simulink model "PlantaSoloActitud"  (Simulink 8.0)
settings: Solver=ode4  StartTime=0.0  StopTime=inf  FixedStep=0.001  RelTol=1e-3
undefined symbols (not defined in the file or in its folder): PlantaActitudOneStepMOD, VEFI_to_VE
libraries: simulink x3
settings Model: Creator=alumno4  LastModifiedBy=David  ExtModeTrigDuration=5000
settings SolverCC: PositivePriorityOrder=on
settings DataIOCC: SignalLoggingSaveFormat=ModelDataLogs
settings OptimizationCC: InlineParams=on
settings DebuggingCC: FcnCallInpInsideContextMsg=UseLocalSettings
settings RTWCC: SystemTargetFile=quarc_windows.tlc  TemplateMakefile=quarc_default_tmf  Description=QUARC Win32 Target  ProcessScript=quarc_windows_make_rtw_hook
settings STFCustomTargetCC: TargetPreCompLibLocation=C:\PROGRA~2\QUARC\lib\2011a\windows\release  CodeReplacementLibrary=ANSI_C  GeneratePreprocessorConditionals=Disable all  SystemTargetFile=quarc_windows.tlc
settings GRTTargetCC: TargetPreCompLibLocation=C:\PROGRA~2\QUARC\lib\2011a\windows\release  ParMdlRefBuildCompliant=off  CompOptLevelCompliant=off  ConcurrentExecutionCompliant=off  CombineOutputUpdateFcns=off  MatFileLogging=off  GRTInterface=on  ExtMode=on  ExtModeMexFile=quarc_comm

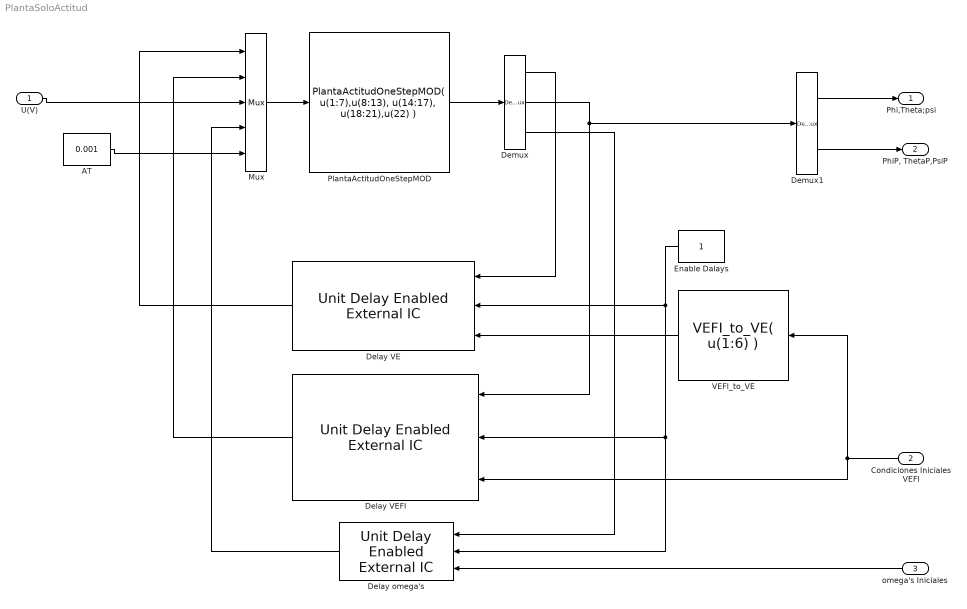
== system PlantaSoloActitud ==
  U(V) : Inport  PortDimensions=[4 1]
  Condiciones Iniciales VEFI : Inport  Port=2  PortDimensions=[6 1]
  omega's Iniciales : Inport  Port=3  PortDimensions=[4 1]
  AT : Constant  Value=0.001  SampleTime=-1
  Delay VE : simulink/Additional Math & Discrete/Additional Discrete/Unit Delay Enabled External IC  tsamp=-1
  Delay VEFI : simulink/Additional Math & Discrete/Additional Discrete/Unit Delay Enabled External IC  tsamp=-1
  Delay omega's : simulink/Additional Math & Discrete/Additional Discrete/Unit Delay Enabled External IC  tsamp=-1
  Demux : Demux  Outputs=[7 6 4]
  Demux1 : Demux  Outputs=[3 3]
  Enable Dalays : Constant
  Mux : Mux  Inputs=5
  PlantaActitudOneStepMOD : MATLABFcn  MATLABFcn="PlantaActitudOneStepMOD( u(1:7),u(8:13), u(14:17), u(18:21),u(22)  )"  OutputDimensions=[17 1]  Output1D=off  SampleTime=0.001
  VEFI_to_VE : MATLABFcn  MATLABFcn=VEFI_to_VE( u(1:6) )  SampleTime=0.001
  Phi,Theta;psi : Outport
  "PhiP, ThetaP,PsiP" : Outport  Port=2
  wires:
  Enable Dalays/1 -> Delay VE/2, Delay VEFI/2, Delay omega's/2
  Delay VE/1 -> Mux/1
  Delay VEFI/1 -> Mux/2
  U(V)/1 -> Mux/3
  omega's Iniciales/1 -> Delay omega's/3
  Delay omega's/1 -> Mux/4
  AT/1 -> Mux/5
  PlantaActitudOneStepMOD/1 -> Demux/1
  Mux/1 -> PlantaActitudOneStepMOD/1
  Demux/3 -> Delay omega's/1
  Demux/2 -> Delay VEFI/1, Demux1/1
  Demux/1 -> Delay VE/1
  Demux1/1 -> Phi,Theta;psi/1
  Demux1/2 -> "PhiP, ThetaP,PsiP"/1
  VEFI_to_VE/1 -> Delay VE/3
  Condiciones Iniciales VEFI/1 -> VEFI_to_VE/1, Delay VEFI/3
